simulink model "BHclientT"  (Simulink 7.4)
settings: Solver=ode3  StartTime=0.0  StopTime=inf  FixedStep=0.005  RelTol=1e-3
libraries: planmant x1
settings Model: Creator=Admin  LastModifiedBy=Admin

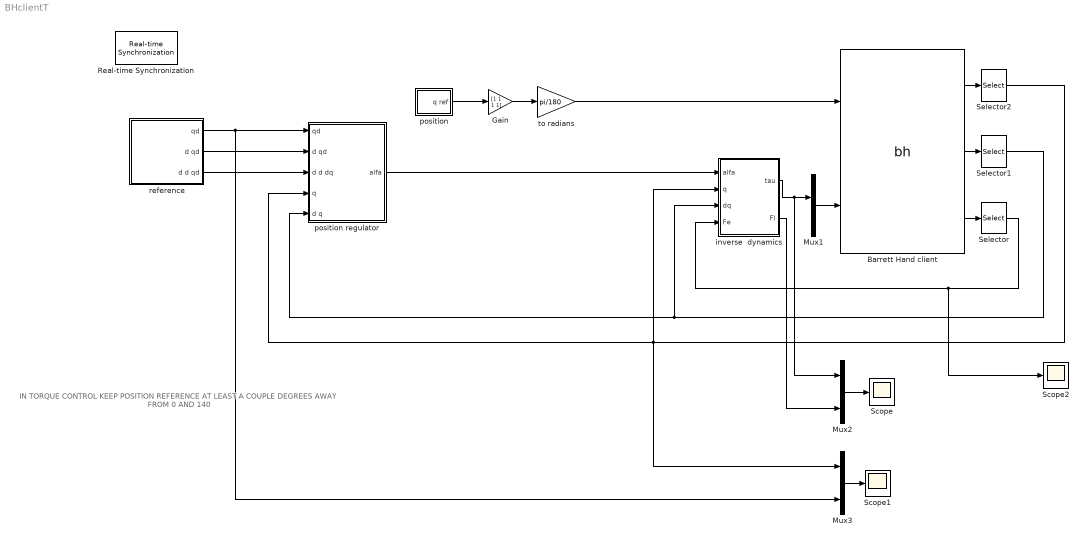
== system BHclientT ==
  note: IN TORQUE CONTROL
      | KEEP POSITION
      | REFERENCE AT
      | LEAST A COUPLE
      | DEGREES AWAY
      | FROM 0 AND 140
  Barrett Hand client : S-Function  FunctionName=bh  Parameters=IP port mode262 mode280 ST a0 a1 a2 a3 a4 a41 a5 a6 a7 a8 a81 a9  EnableBusSupport=off  mask(Barrett Hand UDP client){mode262=Torque, mode280=Torque, IP=193.2.6.168, port=4444, ST=0.005, a0=off, a1=off, a2=off, a3=off, a4=off, a41=off, a5=on, a6=on, a7=off, a8=off, a81=on, a9=off}
      mask prompts: mode262 "BH262 mode"; mode280 "BH280 mode"; port "UDP port"; a0 "Time"; a1 "262 position"; a2 "262 velocity"; a3 "262 deltap"; a4 "262 strain"; a41 "262 strain filt"; a5 "280 position"; a6 "280 velocity"; a7 "280 deltap"; a8 "280 strain"; a81 "280 strain filt"; a9 "pps"
      mask help:
      | Make sure you select the right mode. Sending positions when velocity mode
      | selected may not end well.
      |
      | Units are rad and rad/s. Strain and pps data is raw (no units)
      mask StyleString: popup(Velocity|Position|Torque|Other),popup(Velocity|Position|Torque|Other),edit,edit,edit,checkbox,checkbox,checkbox,checkbox,checkbox,checkbox,checkbox,checkbox,checkbox,checkbox,checkbox,checkbox
      mask CallbackString: togglePorts()|togglePorts()|togglePorts()|togglePorts()||togglePorts()|togglePorts()|togglePorts()|togglePorts()|togglePorts()|togglePorts()|togglePorts()|togglePorts()|togglePorts()|togglePorts()|togglePorts()|togglePorts()
      mask TabNameString: Control,Control,Control,Control,Control,Outputs,Outputs,Outputs,Outputs,Outputs,Outputs,Outputs,Outputs,Outputs,Outputs,Outputs,Outputs
      mask Display: text(0.3, 0.9, '\fontsize{10}IP: {\bf193.2.6.168 \newline\rmport: \bf4444}', 'horizontalAlignment', 'center','texmode','on')color('green') port_label('input',1,'\fontsize{12}BH262 {\newline\bfTorque}','texmode','on')color('green') port_label('input',2,'\fontsize{12}BH280 {\newline\bfTorque}','texmode','on')color('black')port_label('output',1,'\fontsize{11}BH280 {\bfPosition}','texmode','on');port_label('output',2,'BH280 {Velocity}','texmode','on');port_label('output',3,'BH280 {StrainFltr}','texmode','on');
  Gain : Gain  Gain=[1 1 1 1]  ParameterDataType=fixdt(1, 16)  ParameterScaling=2^0  OutDataType=fixdt(1, 16)  OutScaling=2^0
  Mux1 : Mux
  Mux2 : Mux  Inputs=2
  Mux3 : Mux  Inputs=2
  Real-time Synchronization : planmant/Utility/Real-time Synchronization  SystemSampleTime=-1
  Scope : Scope
      settings: YMin=-350  YMax=400
  Scope1 : Scope
      settings: YMin=0.675  YMax=1.175  SaveName=ScopeData2
  Scope2 : Scope
      settings: YMin=-350  YMax=400
  Selector : Selector  InputPortWidth=4  IndexOptions=Index vector (dialog)  Indices=2  OutputSizes=1
  Selector1 : Selector  InputPortWidth=4  IndexOptions=Index vector (dialog)  Indices=2  OutputSizes=1
  Selector2 : Selector  InputPortWidth=4  IndexOptions=Index vector (dialog)  Indices=2  OutputSizes=1
  inverse  dynamics : Stateflow chart
  position : Subsystem
  position regulator : Subsystem  mask{Kp=700, Kd=100}
  reference : Subsystem
  to radians : Gain  Gain=pi/180  ParameterDataType=fixdt(1, 16)  ParameterScaling=2^0  OutDataType=fixdt(1, 16)  OutScaling=2^0
  wires:
  Gain/1 -> to radians/1
  position/1(q ref) -> Gain/1
  to radians/1 -> Barrett Hand client/1
  Mux1/1 -> Barrett Hand client/2
  inverse  dynamics/1(tau) -> Mux1/2, Mux2/1
  Barrett Hand client/2 -> Selector1/1
  Barrett Hand client/1 -> Selector2/1
  Barrett Hand client/3 -> Selector/1
  position regulator/1(alfa) -> inverse  dynamics/1(alfa)
  reference/1(qd) -> position regulator/1(qd), Mux3/2
  reference/2(d qd) -> position regulator/2(d qd)
  reference/3(d d qd) -> position regulator/3(d d dq)
  Selector/1 -> inverse  dynamics/4(Fe), Scope2/1
  Selector1/1 -> inverse  dynamics/3(dq), position regulator/5(d q)
  Selector2/1 -> inverse  dynamics/2(q), position regulator/4(q), Mux3/1
  Mux2/1 -> Scope/1
  inverse  dynamics/2(Fl) -> Mux2/2
  Mux3/1 -> Scope1/1

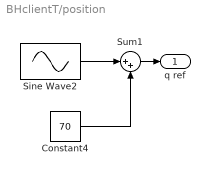
== system BHclientT/position ==
  Constant4 : Constant  Value=70  OutDataType=fixdt(1, 16)  OutScaling=2^0
  Sine Wave2 : Sin  Amplitude=30  Bias=0  Frequency=pi  Phase=pi/4  Samples=10  Offset=0
  Sum1 : Sum  Inputs=|++  OutDataType=fixdt(1, 16)  OutScaling=2^0
  q ref : Outport
  wires:
  Sum1/1 -> q ref/1
  Constant4/1 -> Sum1/2
  Sine Wave2/1 -> Sum1/1

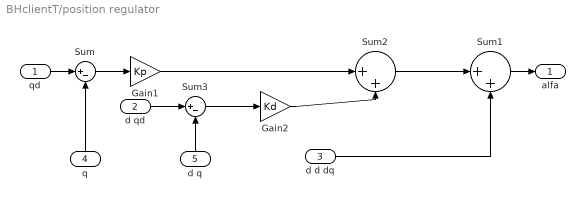
== system BHclientT/position regulator ==
  qd : Inport
  d qd : Inport  Port=2
  d d dq : Inport  Port=3
  q : Inport  Port=4
  d q : Inport  Port=5
  Gain1 : Gain  Gain=Kp  ParameterDataType=fixdt(1, 16)  ParameterScaling=2^0  OutDataType=fixdt(1, 16)  OutScaling=2^0
  Gain2 : Gain  Gain=Kd  ParameterDataType=fixdt(1, 16)  ParameterScaling=2^0  OutDataType=fixdt(1, 16)  OutScaling=2^0
  Sum : Sum  Inputs=|+-  OutDataType=fixdt(1, 16)  OutScaling=2^0
  Sum1 : Sum  Inputs=|++  OutDataType=fixdt(1, 16)  OutScaling=2^0
  Sum2 : Sum  Inputs=|++  OutDataType=fixdt(1, 16)  OutScaling=2^0
  Sum3 : Sum  Inputs=|+-  OutDataType=fixdt(1, 16)  OutScaling=2^0
  alfa : Outport
  wires:
  Sum/1 -> Gain1/1
  Sum3/1 -> Gain2/1
  Gain1/1 -> Sum2/1
  Gain2/1 -> Sum2/2
  Sum2/1 -> Sum1/1
  q/1 -> Sum/2
  d q/1 -> Sum3/2
  qd/1 -> Sum/1
  Sum1/1 -> alfa/1
  d d dq/1 -> Sum1/2
  d qd/1 -> Sum3/1

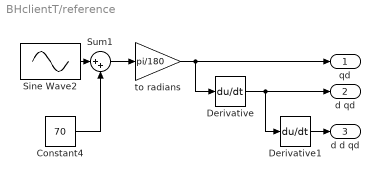
== system BHclientT/reference ==
  Constant4 : Constant  Value=70  OutDataType=fixdt(1, 16)  OutScaling=2^0
  Derivative : Derivative
  Derivative1 : Derivative
  Sine Wave2 : Sin  Amplitude=30  Bias=0  Frequency=0.5*pi  Phase=pi/4  Samples=10  Offset=0
  Sum1 : Sum  Inputs=|++  OutDataType=fixdt(1, 16)  OutScaling=2^0
  to radians : Gain  Gain=pi/180  ParameterDataType=fixdt(1, 16)  ParameterScaling=2^0  OutDataType=fixdt(1, 16)  OutScaling=2^0
  qd : Outport
  d qd : Outport  Port=2
  d d qd : Outport  Port=3
  wires:
  Sum1/1 -> to radians/1
  Constant4/1 -> Sum1/2
  Sine Wave2/1 -> Sum1/1
  Derivative/1 -> d qd/1, Derivative1/1
  Derivative1/1 -> d d qd/1
  to radians/1 -> qd/1, Derivative/1

== matlab function inverse dynamics ==
  data: alfa input double; q input double; dq input double; Fe input double; tau output double; Fl output double
function [tau,Fl] = fcn(alfa,q,dq,Fe)
%#eml
B_q=1;
C_q_dq=0;
F=0.1;
Fl=300*StaticFrictionKoef(dq,alfa);
g_q=0;
Kfe=0;

tau=B_q * alfa + ...    % inertia
    C_q_dq * dq + ...   % coriollis
    F * dq + ...        % friction 
    Fl  + ...           % static friction
    g_q +...            % gravity
    Kfe * Fe;                 % environment

function Fl=StaticFrictionKoef(dq,alfa)
sig=0.4;
KFl=1;

gauss=1/(sig*sqrt(2*pi))*exp(-4*(dq/sig).^2);

Fl=KFl*gauss*sign(alfa);
